simulink subsystem "Bearing_Dynamics"  (R2021b)
settings: Solver=VariableStepAuto  StartTime=0.0  StopTime=10.0  RelTol=1e-3
settings Model: Creator=PhilippSchildt  LastModifiedBy=PhilippSchildt
settings SolverCC: AlgebraicLoopSolver=TrustRegion
settings DebuggingCC: SFMachineParentedDataDiag=warning

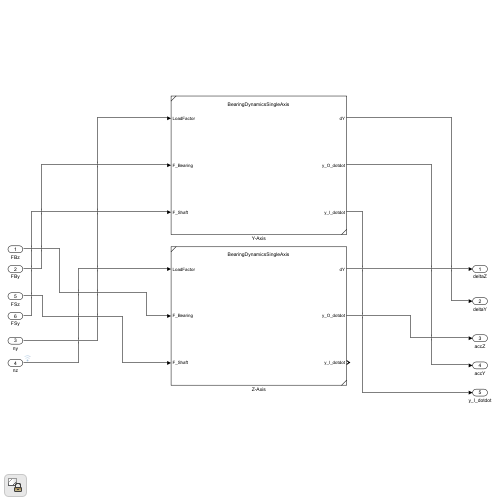
[thumbnail: Simulink's stored preview of the top-level diagram]
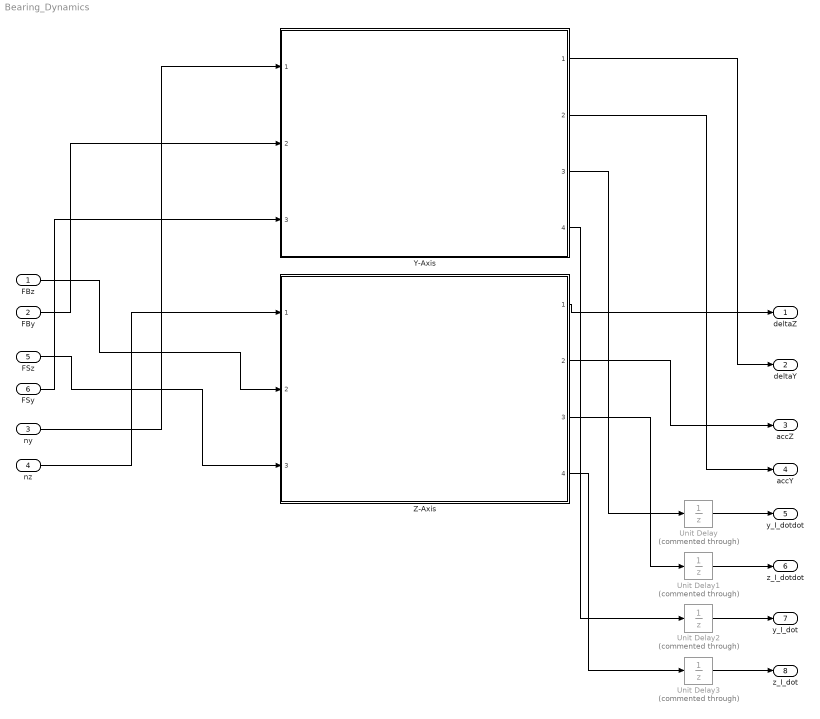
== system Bearing_Dynamics ==
  FBz : Inport
  FBy : Inport  Port=2
  ny : Inport  Port=3
  nz : Inport  Port=4
  FSz : Inport  Port=5
  FSy : Inport  Port=6
  Unit Delay{,1..3} (4 alike) : UnitDelay  Commented=through  SampleTime=-1  HasFrameUpgradeWarning=on
  Y-Axis : Subsystem  ReferencedSubsystem=BearingDynamicsSingleAxis
  Z-Axis : Subsystem  ReferencedSubsystem=BearingDynamicsSingleAxis
  deltaZ : Outport
  deltaY : Outport  Port=2
  accZ : Outport  Port=3
  accY : Outport  Port=4
  y_I_dotdot : Outport  Port=5
  z_I_dotdot : Outport  Port=6
  y_I_dot : Outport  Port=7
  z_I_dot : Outport  Port=8
  wires:
  Y-Axis/1 -> deltaY/1
  ny/1 -> Y-Axis/1
  FBy/1 -> Y-Axis/2
  FSy/1 -> Y-Axis/3
  Y-Axis/2 -> accY/1
  Z-Axis/1 -> deltaZ/1
  Z-Axis/2 -> accZ/1
  nz/1 -> Z-Axis/1
  FBz/1 -> Z-Axis/2
  FSz/1 -> Z-Axis/3
  Y-Axis/3 -> Unit Delay/1
  Z-Axis/3 -> Unit Delay1/1
  Unit Delay1/1 -> z_I_dotdot/1
  Unit Delay/1 -> y_I_dotdot/1
  Unit Delay2/1 -> y_I_dot/1
  Unit Delay3/1 -> z_I_dot/1
  Z-Axis/4 -> Unit Delay3/1
  Y-Axis/4 -> Unit Delay2/1
